simulink model "uz_ParameterID"  (R2021a)
settings: Solver=FixedStepDiscrete  StartTime=0.0  StopTime=160  FixedStep=0.000005  RelTol=1e-3  EnableMultiTasking=on
model workspace (MATLAB code in the model file):
  | cmdLim = Simulink.Parameter;
  | cmdLim.Value = 15;
  | cmdLim.Description = 'Limit for controlling the maximum surface command angle.';
  | cmdLim.Min = 0;
  | cmdLim.Max = 90;
  | cmdLim.DocUnits = 'deg';
  | 
  | dispGain = Simulink.Parameter;
  | dispGain.Value = 0.75;
  | dispGain.Description = 'Gain applied to the displacement error.';
  | dispGain.Min = 0;
  | dispGain.Max = [];
  | dispGain.DocUnits = 'deg/sec/deg';
  | 
  | dispLim = Simulink.Parameter;
  | dispLim.Value = 30;
  | dispLim.Description = 'Limit for controlling the maximum commanded angle.';
  | dispLim.Min = 0;
  | dispLim.Max = 180;
  | dispLim.DocUnits = 'deg';
  | 
  | intGain = Simulink.Parameter;
  | intGain.Value = 0.5;
  | intGain.Description = 'Gain applied to the integral error.';
  | intGain.Min = 0;
  | intGain.Max = [];
  | intGain.DocUnits = 'deg/sec/deg/sec';
  | 
  | intLim = Simulink.Parameter;
  | intLim.Value = 5;
  | intLim.Description = 'Limit for controlling the maximum commanded angle.';
  | intLim.Min = 0;
  | intLim.Max = 90;
  | intLim.DocUnits = 'deg';
  | 
  | rateGain = Simulink.Parameter;
  | rateGain.Value = 2;
  | rateGain.Description = 'Gain applied to the rate error.';
  | rateGain.Min = 0;
  | rateGain.Max = [];
  | rateGain.DocUnits = 'deg/deg/sec';
  | 
  | rateLim = Simulink.Parameter;
  | rateLim.Value = 6;
  | rateLim.Description = 'Limit for controlling the maximum commanded angle.';
  | rateLim.Min = 0;
  | rateLim.Max = 180;
  | rateLim.DocUnits = 'deg/sec';
  | 
  | hdgGain = Simulink.Parameter;
  | hdgGain.Value = 0.015;
values from neighbouring files (symbols this model uses):
  d_d_TMS = 0.005    [Parameter_Init_Buehler_201.m]
  d_f_hardware = 200000    [Parameter_Init_Buehler_201.m]
  d_f_states = 20000    [Parameter_Init_Buehler_201.m]
  d_i_max = 15    [Parameter_Init_Buehler_201.m]
  d_i_min = -d_i_max    (= -15)    [Parameter_Init_Buehler_201.m]
  d_I_n = 8    [Parameter_Init_Buehler_201.m]
  d_J_Coupling_M_E = 2e-6    (= 2e-06)    [Parameter_Init_Buehler_201.m]
  d_J_Coupling_M_Ms = 2e-20    [Parameter_Init_Buehler_201.m]
  d_J_Ms_L = d_J_Ms_M    (= 1.26363648e-05)    [Parameter_Init_Buehler_201.m]
  d_J_Ms_M = 0.5*0.5*((0.5*d_d_Ms)^4)*3.14*d_l_Ms*d_rho_Ms    (= 1.26363648e-05)    [Parameter_Init_Buehler_201.m]
  d_Ki_id = 162.47    [Parameter_Init_Buehler_201.m]
  d_Ki_iq = 162.47    [Parameter_Init_Buehler_201.m]
  d_Ki_n = 1.982    [Parameter_Init_Buehler_201.m]
  d_Kp_id = 0.369    [Parameter_Init_Buehler_201.m]
  d_Kp_iq = 0.369    [Parameter_Init_Buehler_201.m]
  d_Kp_n = 0.198    [Parameter_Init_Buehler_201.m]
  d_L_d = 0.00031    [Parameter_Init_Buehler_201.m]
  d_L_q = 0.00033    [Parameter_Init_Buehler_201.m]
  d_n_n = 3200    [Parameter_Init_Buehler_201.m]
  d_p = 4    [Parameter_Init_Buehler_201.m]
  d_psi_pm = 0.0075    [Parameter_Init_Buehler_201.m]
  d_R_ph = d_R_ph_ph/2    (= 0.089)    [Parameter_Init_Buehler_201.m]
  d_y_max = 10    [Parameter_Init_Buehler_201.m]
  d_y_min = -d_y_max    (= -10)    [Parameter_Init_Buehler_201.m]
undefined symbols (not defined in the file or in its folder): i_dq, i_dq_ref, n_ref, V_abc, v_dq
libraries: fl_lib x47, nesl_utility x30, ee_lib x18, simulink x8, spsabctodq0Lib x2, spsdq0toabcLib x1, spsTriangleGeneratorLib x1
(part 3 of 4)

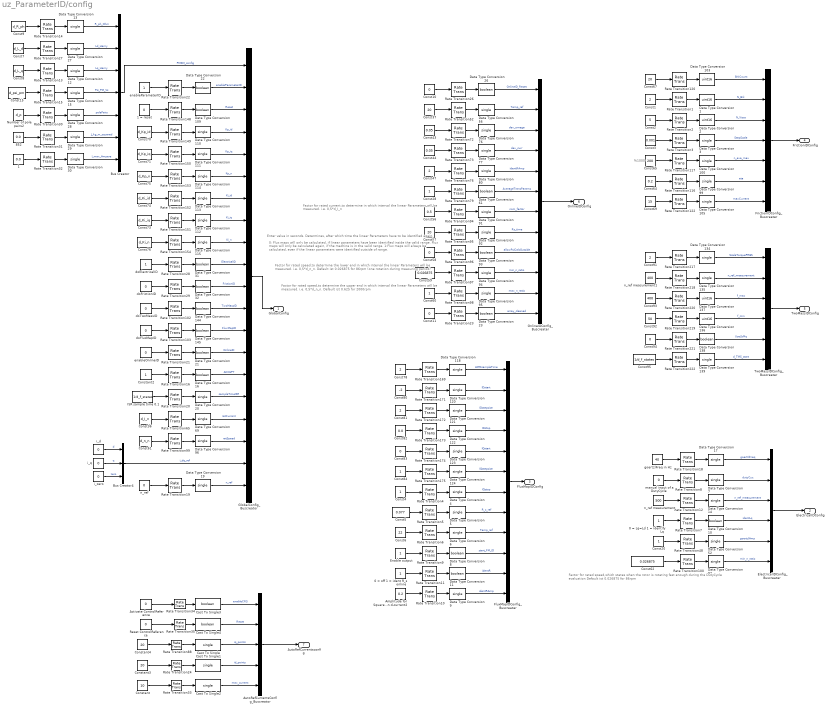
== system uz_ParameterID/config ==
  note: %1000
  note: Factor for rated speed,to determine the upper end in which interval the linear Parameters will
      | be measured. i.e. 0,5*d_n_n.
      | Default ist 0.625 for 2000rpm
  note: 0: Flux maps will only be calculated, if linear parameters have been identified inside the valid range.
      |     Flux maps will only be calculated again, if the machine is in the valid range.
      | 1:Flux maps will always be calculated, even if the linear parameters were identified outside of range.
  note: Enter value in seconds. Determines, after which time the linear Parameters have to be identified again.
  note: Factor for rated current,to determine in which interval the linear Parameters will
      | be measured. i.e. 0,5*d_I_n
  note: Factor for rated speed,to determine the lower end in which interval the linear Parameters will
      | be measured. i.e. 0,5*d_n_n.
      | Default ist 0.026875 for 86rpm (one rotation during measuring period)
  note: Factor for rated speed,which states when the rotor is rotating fast enough during the DutyCycle evaluation
      | Default ist 0.026875 for 86rpm
  "0 = Lq=Ld 1 = identify Lq " : Constant
  0 = off 1 = ident R_s online : Constant
  1 : Constant  Value=0.0
  1 = reset : Constant  Value=0
  852 : Constant  Value=0.0
  Activate ControlReference : Constant  Value=0  OutDataTypeStr=boolean
  Amplitude for SquareWave signal in d-current2 : Constant  Value=0.2
  AutoRefCurrentsConfig_Buscreator : BusCreator  Inputs=5  OutDataTypeStr=Bus: uz_ParaID_AutoRefCurrentsConfig_t
  Bus Creator : BusCreator  Inputs=7  OutDataTypeStr=Bus: uz_PMSM_t
  Bus Creator4 : BusCreator  Inputs=3  OutDataTypeStr=Bus: uz_3ph_dq_t
  Cast To Single : DataTypeConversion  OutDataTypeStr=single
  Cast To Single1 : DataTypeConversion  OutDataTypeStr=single
  Cast To Single2 : DataTypeConversion  OutDataTypeStr=single
  Cast To Single3 : DataTypeConversion  OutDataTypeStr=boolean
  Cast To Single4 : DataTypeConversion  OutDataTypeStr=boolean
  Const{1,47,78,81,91} (5 alike) : Constant  Value=2
  Const{10..11,58,83,94} (5 alike) : Constant  Value=0
  Const15 : Constant  Value=d_psi_pm
  Const2 : Constant  Value=5
  Const{4,20,28,60,84} (5 alike) : Constant
  Const3 : Constant  Value=0.001
  Const36 : Constant  Value=d_I_n
  Const37 : Constant  Value=20
  Const43 : Constant  Value=0.05
  Const44 : Constant  Value=0.05
  Const5 : Constant  Value=0.077
  Const56 : Constant  Value=0.5
  Const57 : Constant  Value=20
  Const59 : Constant  Value=0.026875
  Const6 : Constant  Value=22
  Const61 : Constant  Value=d_n_n
  Const62 : Constant  Value=0.026875
  Const64 : Constant  Value=0.2
  Const65 : Constant  Value=200
  Const67 : Constant  Value=20
  Const69 : Constant  Value=15
  Const7 : Constant  Value=d_L_d
  Const70 : Constant  Value=d_Kp_id
  Const71 : Constant  Value=d_Kp_iq
  Const73 : Constant  Value=d_Ki_iq
  Const74 : Constant  Value=d_Ki_id
  Const75 : Constant  Value=d_Kp_n
  Const76 : Constant  Value=d_Ki_n
  Const8 : Constant  Value=d_L_q
  Const80 : Constant  Value=-2
  Const82 : Constant  Value=0.0
  Const9 : Constant  Value=d_R_ph
  Const92 : Constant  Value=50
  Const93 : Constant  Value=400
  Const95 : Constant  Value=1/d_f_states
  Constant : Constant  Value=10
  Constant2 : Constant
  Constant3 : Constant  Value=20
  Constant4 : Constant  Value=20
  Data Type Conversion{1..2,103,136..137} (5 alike) : DataTypeConversion  OutDataTypeStr=uint16
  Data Type Conversion{8,10..11,16,21..23,26,31..32,61,93,109,138,144..145} (16 alike) : DataTypeConversion  OutDataTypeStr=boolean
  Data Type Conversion{3..7,9,12..15,17,19..20,27..30,52,56,69,76..77,80,91..92,94..97,99..100,105,110..115,118,120..124,134..135,139} (47 alike) : DataTypeConversion  OutDataTypeStr=single
  ElectricalIDConfig_Buscreater : BusCreator  Inputs=6  OutDataTypeStr=Bus: uz_ParaID_ElectricalIDConfig_t
  Enable output : Constant
  FluxMapIDConfig_Buscreater : BusCreator  Inputs=12  OutDataTypeStr=Bus: uz_ParaID_FluxMapIDConfig_t
  FrictionIDConfig_Buscreater : BusCreator  Inputs=7  OutDataTypeStr=Bus: uz_ParaID_FrictionIDConfig_t
  GlobalConfig_Buscreator : BusCreator  Inputs=20  OutDataTypeStr=Bus: uz_ParaID_GlobalConfig_t
  ISR sample time 0.1 : Constant  Value=1/d_f_states
  Number of pole pairs2 : Constant  Value=d_p
  OnlineIDConfig_Buscreater : BusCreator  Inputs=12  OutDataTypeStr=Bus: uz_ParaID_OnlineIDConfig_t
  Rate Transition{1..16,18..24,26..35,48,52,65,72..73,76,79,88,94..100,102..103,116..117,120,122,148..154,169,171..175,217..222} (73 alike) : RateTransition  OutPortSampleTime=1/d_f_states
  Reset ControlReference : Constant  Value=0  OutDataTypeStr=boolean
  TwoMassIDConfig_Buscreater : BusCreator  Inputs=6  OutDataTypeStr=Bus: uz_ParaID_TwoMassIDConfig_t
  doElectricalID : Constant
  doFluxMapID : Constant  Value=0
  doFrictionID : Constant  Value=0
  doTwoMassID : Constant  Value=0
  enableOnlineID : Constant  Value=0
  enableParameterID : Constant
  goertzlFreq in Hz : Constant  Value=40
  i_d : Constant  Value=0  OutDataTypeStr=single
  i_q : Constant  Value=0  OutDataTypeStr=single
  i_zero : Constant  Value=0  OutDataTypeStr=single
  manual input of a DutyCycle : Constant  Value=0
  n_ref : Constant  Value=0
  n_ref measurement : Constant  Value=500
  n_ref measurement1 : Constant  Value=400
  GlobalConfig : Outport
  ElectricalIDConfig : Outport  Port=2
  FluxMapIDConfig : Outport  Port=3
  FrictionIDConfig : Outport  Port=4
  TwoMassIDConfig : Outport  Port=5
  OnlineIDConfig : Outport  Port=6
  AutoRefCurrentsconfig : Outport  Port=7
  wires:
  Data Type Conversion1/1 -> FrictionIDConfig_Buscreater/2  "N_Brk"
  Data Type Conversion99/1 -> FrictionIDConfig_Buscreater/6  "eta"
  Data Type Conversion2/1 -> FrictionIDConfig_Buscreater/3  "N_Visco"
  Data Type Conversion103/1 -> FrictionIDConfig_Buscreater/1  "BrkCount"
  Data Type Conversion105/1 -> FrictionIDConfig_Buscreater/7  "maxCurrent"
  Data Type Conversion100/1 -> FrictionIDConfig_Buscreater/5  "n_eva_max"
  Data Type Conversion3/1 -> FrictionIDConfig_Buscreater/4  "StepScale"
  FrictionIDConfig_Buscreater/1 -> FrictionIDConfig/1
  Rate Transition120/1 -> Data Type Conversion103/1
  Const67/1 -> Rate Transition120/1
  Const1/1 -> Rate Transition1/1
  Rate Transition1/1 -> Data Type Conversion1/1
  Const2/1 -> Rate Transition2/1
  Rate Transition2/1 -> Data Type Conversion2/1
  Const3/1 -> Rate Transition3/1
  Rate Transition3/1 -> Data Type Conversion3/1
  Const65/1 -> Rate Transition117/1
  Const64/1 -> Rate Transition116/1
  Rate Transition116/1 -> Data Type Conversion99/1
  Rate Transition117/1 -> Data Type Conversion100/1
  Const69/1 -> Rate Transition122/1
  Rate Transition122/1 -> Data Type Conversion105/1
  TwoMassIDConfig_Buscreater/1 -> TwoMassIDConfig/1
  Const91/1 -> Rate Transition217/1
  Rate Transition217/1 -> Data Type Conversion134/1
  Data Type Conversion134/1 -> TwoMassIDConfig_Buscreater/1  "ScaleTorquePRBS"
  Rate Transition218/1 -> Data Type Conversion135/1
  n_ref measurement1/1 -> Rate Transition218/1
  Data Type Conversion135/1 -> TwoMassIDConfig_Buscreater/2  "n_ref_measurement"
  Rate Transition219/1 -> Data Type Conversion136/1
  Const93/1 -> Rate Transition220/1
  Const92/1 -> Rate Transition219/1
  Rate Transition220/1 -> Data Type Conversion137/1
  Data Type Conversion137/1 -> TwoMassIDConfig_Buscreater/3  "f_max"
  Data Type Conversion136/1 -> TwoMassIDConfig_Buscreater/4  "f_min"
  Rate Transition221/1 -> Data Type Conversion138/1
  Rate Transition222/1 -> Data Type Conversion139/1
  Const94/1 -> Rate Transition221/1
  Const95/1 -> Rate Transition222/1
  Data Type Conversion138/1 -> TwoMassIDConfig_Buscreater/5  "UseLbMq"
  Data Type Conversion139/1 -> TwoMassIDConfig_Buscreater/6  "d_TMS_start"
  FluxMapIDConfig_Buscreater/1 -> FluxMapIDConfig/1
  Rate Transition172/1 -> Data Type Conversion121/1
  Const80/1 -> Rate Transition171/1
  Const84/1 -> Rate Transition175/1
  Rate Transition175/1 -> Data Type Conversion124/1
  Rate Transition171/1 -> Data Type Conversion120/1
  Rate Transition174/1 -> Data Type Conversion123/1
  Const78/1 -> Rate Transition169/1
  Const82/1 -> Rate Transition173/1
  Const81/1 -> Rate Transition172/1
  Rate Transition169/1 -> Data Type Conversion118/1
  Rate Transition173/1 -> Data Type Conversion122/1
  Const83/1 -> Rate Transition174/1
  Data Type Conversion118/1 -> FluxMapIDConfig_Buscreater/1  "AMMsampleTime"
  Data Type Conversion120/1 -> FluxMapIDConfig_Buscreater/2  "IDstart"
  Rate Transition5/1 -> Data Type Conversion5/1
  Rate Transition6/1 -> Data Type Conversion6/1
  Const6/1 -> Rate Transition6/1
  Const4/1 -> Rate Transition4/1
  Const5/1 -> Rate Transition5/1
  Rate Transition4/1 -> Data Type Conversion4/1
  Data Type Conversion121/1 -> FluxMapIDConfig_Buscreater/3  "IDstepsize"
  Data Type Conversion122/1 -> FluxMapIDConfig_Buscreater/4  "IDstop"
  Data Type Conversion123/1 -> FluxMapIDConfig_Buscreater/5  "IQstart"
  Data Type Conversion124/1 -> FluxMapIDConfig_Buscreater/6  "IQstepsize"
  Data Type Conversion4/1 -> FluxMapIDConfig_Buscreater/7  "IQstop"
  Data Type Conversion5/1 -> FluxMapIDConfig_Buscreater/8  "R_s_ref"
  Data Type Conversion6/1 -> FluxMapIDConfig_Buscreater/9  "Temp_ref"
  ElectricalIDConfig_Buscreater/1 -> ElectricalIDConfig/1
  OnlineIDConfig_Buscreater/1 -> OnlineIDConfig/1
  Const37/1 -> Rate Transition52/1
  Rate Transition52/1 -> Data Type Conversion56/1
  Data Type Conversion56/1 -> OnlineIDConfig_Buscreater/2  "Temp_ref"
  Data Type Conversion77/1 -> OnlineIDConfig_Buscreater/4  "dev_curr"
  Data Type Conversion76/1 -> OnlineIDConfig_Buscreater/3  "dev_omega"
  Const44/1 -> Rate Transition73/1
  Const43/1 -> Rate Transition72/1
  Rate Transition72/1 -> Data Type Conversion76/1
  Const47/1 -> Rate Transition76/1
  Rate Transition73/1 -> Data Type Conversion77/1
  Rate Transition76/1 -> Data Type Conversion80/1
  Data Type Conversion80/1 -> OnlineIDConfig_Buscreater/5  "identRAmp"
  Data Type Conversion61/1 -> OnlineIDConfig_Buscreater/6  "AverageTransParams"
  Const28/1 -> Rate Transition79/1
  Rate Transition79/1 -> Data Type Conversion61/1
  Const56/1 -> Rate Transition94/1
  Data Type Conversion93/1 -> OnlineIDConfig_Buscreater/9  "allowPsiCalcOutside"
  Rate Transition94/1 -> Data Type Conversion91/1
  Data Type Conversion95/1 -> OnlineIDConfig_Buscreater/11  "max_n_ratio"
  Const58/1 -> Rate Transition96/1
  Const57/1 -> Rate Transition95/1
  Data Type Conversion91/1 -> OnlineIDConfig_Buscreater/7  "nom_factor"
  Rate Transition98/1 -> Data Type Conversion95/1
  Data Type Conversion92/1 -> OnlineIDConfig_Buscreater/8  "Rs_time"
  Rate Transition96/1 -> Data Type Conversion93/1
  Const59/1 -> Rate Transition97/1
  Rate Transition97/1 -> Data Type Conversion94/1
  Const60/1 -> Rate Transition98/1
  Data Type Conversion94/1 -> OnlineIDConfig_Buscreater/10  "min_n_ratio"
  Rate Transition95/1 -> Data Type Conversion92/1
  1 = reset/1 -> Rate Transition148/1
  Rate Transition149/1 -> Data Type Conversion110/1
  Const75/1 -> Rate Transition153/1
  Rate Transition150/1 -> Data Type Conversion111/1
  Rate Transition152/1 -> Data Type Conversion113/1
  Const71/1 -> Rate Transition150/1
  Rate Transition154/1 -> Data Type Conversion115/1
  Const76/1 -> Rate Transition154/1
  Rate Transition148/1 -> Data Type Conversion109/1
  Const70/1 -> Rate Transition149/1
  Rate Transition153/1 -> Data Type Conversion114/1
  Const73/1 -> Rate Transition151/1
  Rate Transition151/1 -> Data Type Conversion112/1
  Const74/1 -> Rate Transition152/1
  Data Type Conversion109/1 -> GlobalConfig_Buscreator/3  "Reset"
  Data Type Conversion110/1 -> GlobalConfig_Buscreator/4  "Kp_id"
  Data Type Conversion111/1 -> GlobalConfig_Buscreator/5  "Kp_iq"
  Data Type Conversion114/1 -> GlobalConfig_Buscreator/6  "Kp_n"
  Data Type Conversion113/1 -> GlobalConfig_Buscreator/7  "Ki_id"
  Data Type Conversion112/1 -> GlobalConfig_Buscreator/8  "Ki_iq"
  Data Type Conversion115/1 -> GlobalConfig_Buscreator/9  "Ki_n"
  Rate Transition28/1 -> Data Type Conversion31/1
  Data Type Conversion32/1 -> GlobalConfig_Buscreator/11  "FrictionID"
  doTwoMassID/1 -> Rate Transition102/1
  Data Type Conversion145/1 -> GlobalConfig_Buscreator/13  "FluxMapID"
  Rate Transition29/1 -> Data Type Conversion32/1
  doFluxMapID/1 -> Rate Transition103/1
  Rate Transition103/1 -> Data Type Conversion145/1
  Data Type Conversion31/1 -> GlobalConfig_Buscreator/10  "ElectricalID"
  Rate Transition102/1 -> Data Type Conversion144/1
  doElectricalID/1 -> Rate Transition28/1
  Data Type Conversion144/1 -> GlobalConfig_Buscreator/12  "TwoMassID"
  doFrictionID/1 -> Rate Transition29/1
  Constant2/1 -> Rate Transition16/1
  Rate Transition16/1 -> Data Type Conversion16/1
  Data Type Conversion16/1 -> GlobalConfig_Buscreator/15  "ACCEPT"
  ISR sample time 0.1/1 -> Rate Transition20/1
  Rate Transition20/1 -> Data Type Conversion20/1
  Const36/1 -> Rate Transition65/1
  Const61/1 -> Rate Transition99/1
  Rate Transition99/1 -> Data Type Conversion96/1
  Rate Transition65/1 -> Data Type Conversion69/1
  Data Type Conversion69/1 -> GlobalConfig_Buscreator/17  "ratCurrent"
  Data Type Conversion96/1 -> GlobalConfig_Buscreator/18  "ratSpeed"
  enableOnlineID/1 -> Rate Transition21/1
  Data Type Conversion21/1 -> GlobalConfig_Buscreator/14  "OnlineID"
  Rate Transition21/1 -> Data Type Conversion21/1
  GlobalConfig_Buscreator/1 -> GlobalConfig/1
  Rate Transition26/1 -> Data Type Conversion26/1
  Data Type Conversion26/1 -> OnlineIDConfig_Buscreater/1  "OnlineID_Reset"
  Const10/1 -> Rate Transition26/1
  Data Type Conversion11/1 -> FluxMapIDConfig_Buscreater/11  "identR"
  0 = off 1 = ident R_s online/1 -> Rate Transition11/1
  Rate Transition10/1 -> Data Type Conversion9/1
  Amplitude for SquareWave signal in d-current2/1 -> Rate Transition10/1
  Data Type Conversion9/1 -> FluxMapIDConfig_Buscreater/12  "identRAmp"
  Rate Transition11/1 -> Data Type Conversion11/1
  Data Type Conversion8/1 -> FluxMapIDConfig_Buscreater/10  "start_FM_ID"
  Rate Transition9/1 -> Data Type Conversion8/1
  Enable output/1 -> Rate Transition9/1
  Bus Creator/1 -> GlobalConfig_Buscreator/1  "PMSM_config"
  Const15/1 -> Rate Transition15/1
  Rate Transition15/1 -> Data Type Conversion15/1
  Data Type Conversion15/1 -> Bus Creator/4  "Psi_PM_Vs"
  Rate Transition30/1 -> Data Type Conversion28/1
  Number of pole pairs2/1 -> Rate Transition30/1
  Data Type Conversion28/1 -> Bus Creator/5  "polePairs"
  Rate Transition31/1 -> Data Type Conversion29/1
  852/1 -> Rate Transition31/1
  Data Type Conversion29/1 -> Bus Creator/6  "J_kg_m_squared"
  Rate Transition32/1 -> Data Type Conversion30/1
  1/1 -> Rate Transition32/1
  Data Type Conversion30/1 -> Bus Creator/7  "I_max_Ampere"
  Data Type Conversion13/1 -> Bus Creator/1  "R_ph_Ohm"
  Const9/1 -> Rate Transition14/1
  Rate Transition14/1 -> Data Type Conversion13/1
  Data Type Conversion27/1 -> Bus Creator/2  "Ld_Henry"
  Rate Transition13/1 -> Data Type Conversion12/1
  Rate Transition27/1 -> Data Type Conversion27/1
  Data Type Conversion12/1 -> Bus Creator/3  "Lq_Henry"
  Const7/1 -> Rate Transition27/1
  Const8/1 -> Rate Transition13/1
  i_q/1 -> Bus Creator4/2  "q"
  i_d/1 -> Bus Creator4/1  "d"
  i_zero/1 -> Bus Creator4/3  "zero"
  Bus Creator4/1 -> GlobalConfig_Buscreator/19  "i_dq_ref"
  Rate Transition19/1 -> Data Type Conversion19/1
  n_ref/1 -> Rate Transition19/1
  Data Type Conversion19/1 -> GlobalConfig_Buscreator/20  "n_ref"
  enableParameterID/1 -> Rate Transition22/1
  Rate Transition22/1 -> Data Type Conversion22/1
  Data Type Conversion22/1 -> GlobalConfig_Buscreator/2  "enableParameterID"
  Rate Transition23/1 -> Data Type Conversion23/1
  Const11/1 -> Rate Transition23/1
  Data Type Conversion23/1 -> OnlineIDConfig_Buscreater/12  "array_cleaned"
  Constant4/1 -> Rate Transition88/1
  Rate Transition88/1 -> Cast To Single/1
  Rate Transition24/1 -> Cast To Single1/1
  Constant3/1 -> Rate Transition24/1
  Rate Transition33/1 -> Cast To Single2/1
  Constant/1 -> Rate Transition33/1
  Rate Transition34/1 -> Cast To Single3/1
  Cast To Single3/1 -> AutoRefCurrentsConfig_Buscreator/1  "enableCRS"
  Activate ControlReference/1 -> Rate Transition34/1
  Rate Transition35/1 -> Cast To Single4/1
  Reset ControlReference/1 -> Rate Transition35/1
  Cast To Single4/1 -> AutoRefCurrentsConfig_Buscreator/2  "Reset"
  Cast To Single/1 -> AutoRefCurrentsConfig_Buscreator/3  "iq_points"
  Cast To Single1/1 -> AutoRefCurrentsConfig_Buscreator/4  "id_points"
  Cast To Single2/1 -> AutoRefCurrentsConfig_Buscreator/5  "max_current"
  AutoRefCurrentsConfig_Buscreator/1 -> AutoRefCurrentsconfig/1
  Data Type Conversion20/1 -> GlobalConfig_Buscreator/16  "sampleTimeISR"
  Rate Transition18/1 -> Data Type Conversion17/1
  Data Type Conversion17/1 -> ElectricalIDConfig_Buscreater/1  "goertzlFreq"
  goertzlFreq in Hz/1 -> Rate Transition18/1
  Rate Transition8/1 -> Data Type Conversion7/1
  Const20/1 -> Rate Transition48/1
  Data Type Conversion14/1 -> ElectricalIDConfig_Buscreater/3  "n_ref_measurement"
  manual input of a DutyCycle/1 -> Rate Transition8/1
  "0 = Lq=Ld 1 = identify Lq "/1 -> Rate Transition7/1
  Const62/1 -> Rate Transition100/1
  n_ref measurement/1 -> Rate Transition12/1
  Data Type Conversion7/1 -> ElectricalIDConfig_Buscreater/2  "dutyCyc"
  Data Type Conversion97/1 -> ElectricalIDConfig_Buscreater/6  "min_n_ratio"
  Rate Transition7/1 -> Data Type Conversion10/1
  Rate Transition48/1 -> Data Type Conversion52/1
  Rate Transition12/1 -> Data Type Conversion14/1
  Data Type Conversion52/1 -> ElectricalIDConfig_Buscreater/5  "goertzlAmp"
  Data Type Conversion10/1 -> ElectricalIDConfig_Buscreater/4  "identLq"
  Rate Transition100/1 -> Data Type Conversion97/1

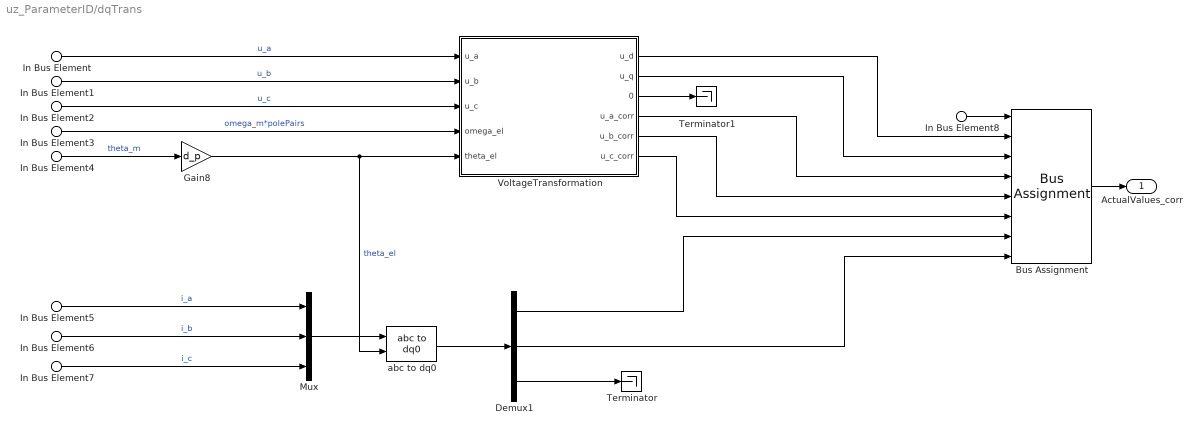
== system uz_ParameterID/dqTrans ==
  In Bus Element8 : Inport  PortName=ActualValues
  In Bus Element3 : Inport  PortName=ActualValues  Element=omega_el
  In Bus Element4 : Inport  PortName=ActualValues  Element=theta_m
  In Bus Element : Inport  PortName=ActualValues  Element=V_abc.a
  In Bus Element1 : Inport  PortName=ActualValues  Element=V_abc.b
  In Bus Element2 : Inport  PortName=ActualValues  Element=V_abc.c
  In Bus Element5 : Inport  PortName=ActualValues  Element=I_abc.a
  In Bus Element6 : Inport  PortName=ActualValues  Element=I_abc.b
  In Bus Element7 : Inport  PortName=ActualValues  Element=I_abc.c
  Bus Assignment : BusAssignment  AssignedSignals=v_dq.d,v_dq.q,V_abc.a,V_abc.b,V_abc.c,i_dq.d,i_dq.q
  Demux1 : Demux  Outputs=3
  Gain8 : Gain  Gain=d_p  OutDataTypeStr=single
  Mux : Mux  Inputs=3
  Terminator : Terminator
  Terminator1 : Terminator
  VoltageTransformation : Subsystem
  abc to dq0 : spsabctodq0Lib/abc to dq0  Alignment=Aligned with phase A axis
  ActualValues_corr : Outport  OutDataTypeStr=Bus: uz_ParaID_ActualValues_t
  wires:
  VoltageTransformation/3(0) -> Terminator1/1
  In Bus Element3/1 -> VoltageTransformation/4(omega_el)  "omega_m*polePairs"
  In Bus Element2/1 -> VoltageTransformation/3(u_c)  "u_c"
  In Bus Element1/1 -> VoltageTransformation/2(u_b)  "u_b"
  In Bus Element/1 -> VoltageTransformation/1(u_a)  "u_a"
  Demux1/3 -> Terminator/1
  Mux/1 -> abc to dq0/1
  In Bus Element7/1 -> Mux/3  "i_c"
  In Bus Element6/1 -> Mux/2  "i_b"
  In Bus Element5/1 -> Mux/1  "i_a"
  Demux1/2 -> Bus Assignment/8
  Demux1/1 -> Bus Assignment/7
  abc to dq0/1 -> Demux1/1
  VoltageTransformation/2(u_q) -> Bus Assignment/3
  VoltageTransformation/1(u_d) -> Bus Assignment/2
  VoltageTransformation/4(u_a_corr) -> Bus Assignment/4
  VoltageTransformation/5(u_b_corr) -> Bus Assignment/5
  VoltageTransformation/6(u_c_corr) -> Bus Assignment/6
  In Bus Element8/1 -> Bus Assignment/1
  Bus Assignment/1 -> ActualValues_corr/1
  Gain8/1 -> abc to dq0/2, VoltageTransformation/5(theta_el)  "theta_el"
  In Bus Element4/1 -> Gain8/1  "theta_m"

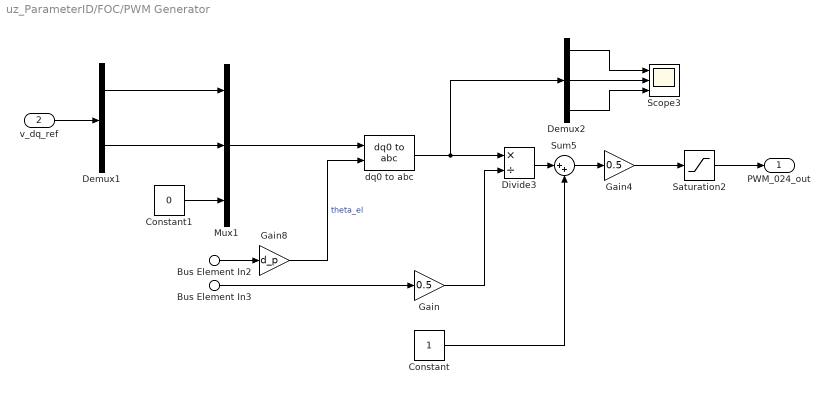
== system uz_ParameterID/FOC/PWM Generator ==
  Bus Element In2 : Inport  PortName=ActualValues  Element=theta_m
  Bus Element In3 : Inport  PortName=ActualValues  Element=V_DC
  v_dq_ref : Inport  Port=2
  Constant : Constant  OutDataTypeStr=single
  Constant1 : Constant  Value=0  OutDataTypeStr=single
  Demux1 : Demux  Outputs=2
  Demux2 : Demux  Outputs=3
  Divide3 : Product  Inputs=*/
  Gain : Gain  Gain=0.5
  Gain4 : Gain  Gain=0.5
  Gain8 : Gain  Gain=d_p  OutDataTypeStr=single
  Mux1 : Mux  Inputs=3
  Saturation2 : Saturate  UpperLimit=1  LowerLimit=0
  Scope3 : Scope  NumInputPorts=3
  Sum5 : Sum  Inputs=|++
  dq0 to abc : spsdq0toabcLib/dq0 to abc  Alignment=Aligned with phase A axis
  PWM_024_out : Outport  VectorParamsAs1DForOutWhenUnconnected=off
  wires:
  Constant/1 -> Sum5/2
  Demux2/2 -> Scope3/2
  Gain4/1 -> Saturation2/1
  Demux2/1 -> Scope3/1
  Demux2/3 -> Scope3/3
  Gain/1 -> Divide3/2
  Sum5/1 -> Gain4/1
  Mux1/1 -> dq0 to abc/1
  dq0 to abc/1 -> Demux2/1, Divide3/1
  Divide3/1 -> Sum5/1
  Bus Element In3/1 -> Gain/1
  Constant1/1 -> Mux1/3
  Demux1/2 -> Mux1/2
  Saturation2/1 -> PWM_024_out/1
  v_dq_ref/1 -> Demux1/1
  Demux1/1 -> Mux1/1
  Bus Element In2/1 -> Gain8/1
  Gain8/1 -> dq0 to abc/2  "theta_el"

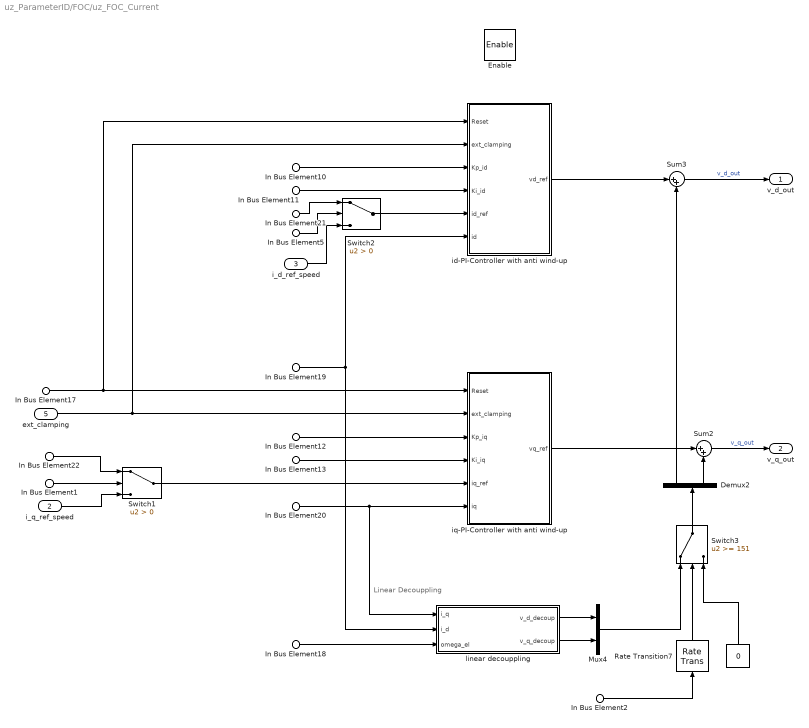
== system uz_ParameterID/FOC/uz_FOC_Current ==
  note: Linear Decouppling
  In Bus Element18 : Inport  PortName=ActualValues  Element=omega_el
  In Bus Element19 : Inport  PortName=ActualValues  Element=i_dq.d
  In Bus Element20 : Inport  PortName=ActualValues  Element=i_dq.q
  i_q_ref_speed : Inport  Port=2
  i_d_ref_speed : Inport  Port=3
  In Bus Element17 : Inport  Port=4  PortName=FOC_State_outputs  Element=resetIntegrator
  In Bus Element11 : Inport  Port=4  PortName=FOC_State_outputs  Element=Ki_id_out
  In Bus Element10 : Inport  Port=4  PortName=FOC_State_outputs  Element=Kp_id_out
  In Bus Element12 : Inport  Port=4  PortName=FOC_State_outputs  Element=Kp_iq_out
  In Bus Element13 : Inport  Port=4  PortName=FOC_State_outputs  Element=Ki_iq_out
  In Bus Element1 : Inport  Port=4  PortName=FOC_State_outputs  Element=enableFOC_current
  In Bus Element5 : Inport  Port=4  PortName=FOC_State_outputs  Element=enableFOC_current
  In Bus Element2 : Inport  Port=4  PortName=FOC_State_outputs  Element=activeState
  In Bus Element21 : Inport  Port=4  PortName=FOC_State_outputs  Element=i_dq_ref.d
  In Bus Element22 : Inport  Port=4  PortName=FOC_State_outputs  Element=i_dq_ref.q
  ext_clamping : Inport  Port=5
  Enable : EnablePort
  " " : Constant  Value=0  OutDataTypeStr=single
  Demux2 : Demux  Outputs=2
  Mux4 : Mux  Inputs=2
  Rate Transition7 : RateTransition  OutPortSampleTime=1/d_f_hardware
  Sum2 : Sum  Inputs=|++
  Sum3 : Sum  Inputs=|++
  Switch1 : Switch  Criteria=u2 > Threshold
  Switch2 : Switch  Criteria=u2 > Threshold
  Switch3 : Switch  Threshold=151
  id-PI-Controller with anti wind-up : Subsystem
  iq-PI-Controller with anti wind-up : Subsystem
  linear decouppling : Subsystem
  v_d_out : Outport
  v_q_out : Outport  Port=2
  wires:
  In Bus Element22/1 -> Switch1/1
  In Bus Element1/1 -> Switch1/2
  Demux2/2 -> Sum2/2
  id-PI-Controller with anti wind-up/1(vd_ref) -> Sum3/1
  In Bus Element19/1 -> id-PI-Controller with anti wind-up/6(id), linear decouppling/2(i_d)
  Demux2/1 -> Sum3/2
  linear decouppling/2(v_q_decoup) -> Mux4/2
  linear decouppling/1(v_d_decoup) -> Mux4/1
  ext_clamping/1 -> iq-PI-Controller with anti wind-up/2(ext_clamping), id-PI-Controller with anti wind-up/2(ext_clamping)
  Switch1/1 -> iq-PI-Controller with anti wind-up/5(iq_ref)
  Sum3/1 -> v_d_out/1  "v_d_out"
  In Bus Element10/1 -> id-PI-Controller with anti wind-up/3(Kp_id)
  In Bus Element18/1 -> linear decouppling/3(omega_el)
  In Bus Element17/1 -> iq-PI-Controller with anti wind-up/1(Reset), id-PI-Controller with anti wind-up/1(Reset)
  In Bus Element12/1 -> iq-PI-Controller with anti wind-up/3(Kp_iq)
  i_q_ref_speed/1 -> Switch1/3
  iq-PI-Controller with anti wind-up/1(vq_ref) -> Sum2/1
  In Bus Element20/1 -> linear decouppling/1(i_q), iq-PI-Controller with anti wind-up/6(iq)
  i_d_ref_speed/1 -> Switch2/3
  In Bus Element21/1 -> Switch2/1
  Switch2/1 -> id-PI-Controller with anti wind-up/5(id_ref)
  In Bus Element5/1 -> Switch2/2
  Mux4/1 -> Switch3/1
  In Bus Element13/1 -> iq-PI-Controller with anti wind-up/4(Ki_iq)
  In Bus Element11/1 -> id-PI-Controller with anti wind-up/4(Ki_id)
  Sum2/1 -> v_q_out/1  "v_q_out"
  In Bus Element2/1 -> Rate Transition7/1
  Rate Transition7/1 -> Switch3/2
  Switch3/1 -> Demux2/1
  " "/1 -> Switch3/3

== system uz_ParameterID/FOC/uz_FOC_Speed ==
  In Bus Element18 : Inport  PortName=ActualValues  Element=omega_el
  In Bus Element19 : Inport  PortName=ActualValues  Element=V_DC
  In Bus Element : Inport  Port=2  PortName=TwoMassID_output  Element=PRBS_out
  In Bus Element13 : Inport  Port=3  PortName=FOC_State_outputs  Element=Kp_n_out
  In Bus Element14 : Inport  Port=3  PortName=FOC_State_outputs  Element=Ki_n_out
  In Bus Element15 : Inport  Port=3  PortName=FOC_State_outputs  Element=n_ref_FOC
  In Bus Element5 : Inport  Port=3  PortName=FOC_State_outputs  Element=resetIntegrator
  In Bus Element21 : Inport  Port=3  PortName=FOC_State_outputs  Element=i_dq_ref.d
  ext_clamping : Inport  Port=4
  Enable : EnablePort
  Field Weakening : Subsystem
  Sum5 : Sum  Inputs=|++
  omega-PI-Controller with anti wind-up : Subsystem
  i_q_ref : Outport  OutDataTypeStr=single
  id_soll : Outport  Port=2  OutDataTypeStr=single
  wires:
  In Bus Element/1 -> Sum5/2  "PRBS Excitation"
  In Bus Element21/1 -> Field Weakening/3(id_ref_input)
  In Bus Element13/1 -> omega-PI-Controller with anti wind-up/3(Kp_n)
  Field Weakening/2(id_Soll) -> id_soll/1
  In Bus Element19/1 -> Field Weakening/2(V_DC)
  ext_clamping/1 -> omega-PI-Controller with anti wind-up/2(ext_clamping)
  In Bus Element18/1 -> Field Weakening/1(omega_el), omega-PI-Controller with anti wind-up/6(omega)
  In Bus Element14/1 -> omega-PI-Controller with anti wind-up/4(Ki_n)
  In Bus Element15/1 -> omega-PI-Controller with anti wind-up/5(n_ref_rpm)
  In Bus Element5/1 -> omega-PI-Controller with anti wind-up/1(Reset)
  omega-PI-Controller with anti wind-up/1(iq_ref) -> Sum5/1
  Sum5/1 -> i_q_ref/1
  Field Weakening/1(iq_max) -> omega-PI-Controller with anti wind-up/7(iq_max)

== system uz_ParameterID/Hardware/Coupling Encoder ==
  note: 1) Add Subsystem or Model blocks as valid variant choices.
      | 2) You cannot connect blocks at this level. At simulation, connectivity is automatically
      | determined, based on the active variant and port name matching.
  Inertia : Subsystem  VariantControl=(default)
  Spring Damper System : Subsystem  VariantControl=TMS1
  Input : PMIOPort  Side=Left
  output : PMIOPort  Port=2  Side=Right

== system uz_ParameterID/Hardware/Measurement Shaft ==
  note: 1) Add Subsystem or Model blocks as valid variant choices.
      | 2) You cannot connect blocks at this level. At simulation, connectivity is automatically
      | determined, based on the active variant and port name matching.
  Spring Damper System : Subsystem  VariantControl=TMS1
  default : Subsystem  VariantControl=(default)
  Input : PMIOPort  Side=Left
  output : PMIOPort  Port=2  Side=Right

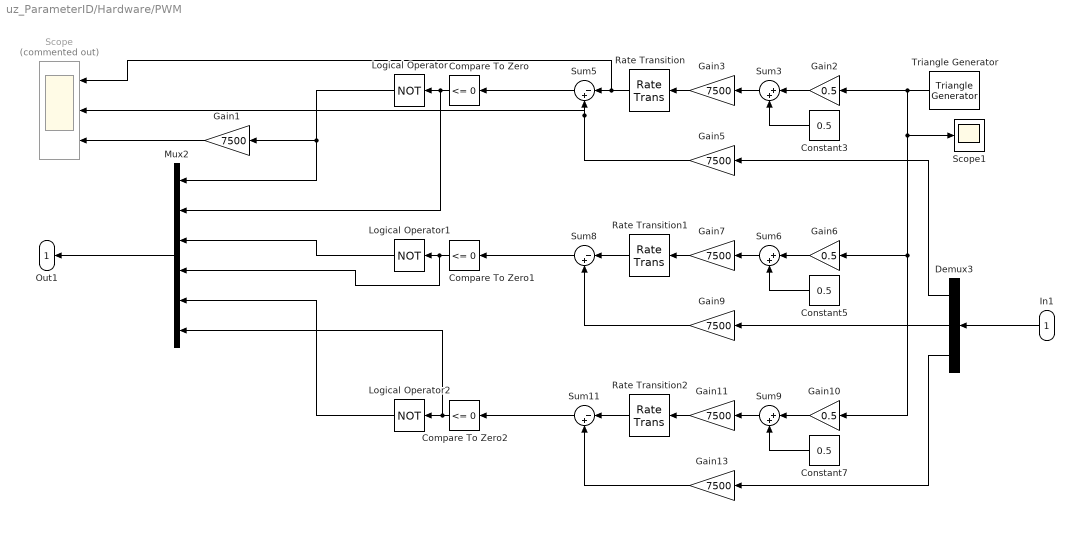
== system uz_ParameterID/Hardware/PWM ==
  In1 : Inport
  Compare To Zero : simulink/Logic and Bit Operations/Compare To Zero  relop=<=  OutDataTypeStr=boolean
  Compare To Zero1 : simulink/Logic and Bit Operations/Compare To Zero  relop=<=  OutDataTypeStr=boolean
  Compare To Zero2 : simulink/Logic and Bit Operations/Compare To Zero  relop=<=  OutDataTypeStr=boolean
  Constant3 : Constant  Value=0.5
  Constant5 : Constant  Value=0.5
  Constant7 : Constant  Value=0.5
  Demux3 : Demux  Outputs=3
  Gain{1,3,5,7,9,11,13} (7 alike) : Gain  Gain=7500  ParamDataTypeStr=single
  Gain10 : Gain  Gain=0.5
  Gain2 : Gain  Gain=0.5
  Gain6 : Gain  Gain=0.5
  Logical Operator : Logic  Operator=NOT  AllPortsSameDT=off  OutDataTypeStr=boolean
  Logical Operator1 : Logic  Operator=NOT  AllPortsSameDT=off  OutDataTypeStr=boolean
  Logical Operator2 : Logic  Operator=NOT  AllPortsSameDT=off  OutDataTypeStr=boolean
  Mux2 : Mux  Inputs=6
  Rate Transition : RateTransition  OutPortSampleTime=1/d_f_hardware
  Rate Transition1 : RateTransition  OutPortSampleTime=1/d_f_hardware
  Rate Transition2 : RateTransition  OutPortSampleTime=1/d_f_hardware
  Scope : Scope  Commented=on  NumInputPorts=3
  Scope1 : Scope
  Sum11 : Sum  Inputs=|-+
  Sum3 : Sum  Inputs=|++
  Sum5 : Sum  Inputs=|-+
  Sum6 : Sum  Inputs=|++
  Sum8 : Sum  Inputs=|-+
  Sum9 : Sum  Inputs=|++
  Triangle Generator : spsTriangleGeneratorLib/Triangle Generator  Freq=10000  Phase=0  Ts=0
  Out1 : Outport  VectorParamsAs1DForOutWhenUnconnected=off
  wires:
  Demux3/3 -> Gain13/1
  Logical Operator2/1 -> Mux2/5
  Logical Operator1/1 -> Mux2/3
  Mux2/1 -> Out1/1
  Compare To Zero2/1 -> Mux2/6, Logical Operator2/1
  Gain10/1 -> Sum9/1
  Sum8/1 -> Compare To Zero1/1
  Gain6/1 -> Sum6/1
  Sum9/1 -> Gain11/1
  Triangle Generator/1 -> Scope1/1, Gain10/1, Gain6/1, Gain2/1
  Sum6/1 -> Gain7/1
  Demux3/2 -> Gain9/1
  Compare To Zero1/1 -> Mux2/4, Logical Operator1/1
  Constant5/1 -> Sum6/2
  Constant7/1 -> Sum9/2
  Sum11/1 -> Compare To Zero2/1
  Sum3/1 -> Gain3/1
  Constant3/1 -> Sum3/2
  Demux3/1 -> Gain5/1
  Sum5/1 -> Compare To Zero/1
  Gain2/1 -> Sum3/1
  In1/1 -> Demux3/1
  Gain3/1 -> Rate Transition/1
  Gain7/1 -> Rate Transition1/1
  Gain11/1 -> Rate Transition2/1
  Gain5/1 -> Scope/2, Sum5/2
  Gain9/1 -> Sum8/2
  Gain13/1 -> Sum11/2
  Rate Transition/1 -> Scope/1, Sum5/1
  Rate Transition1/1 -> Sum8/1
  Rate Transition2/1 -> Sum11/1
  Logical Operator/1 -> Gain1/1, Mux2/1
  Compare To Zero/1 -> Mux2/2, Logical Operator/1
  Gain1/1 -> Scope/3

== system uz_ParameterID/Hardware/Switch f. TMS ==
  note: 1) Add Subsystem or Model blocks as valid variant choices.
      | 2) You cannot connect blocks at this level. At simulation, connectivity is automatically
      | determined, based on the active variant and port name matching.
  closed : Subsystem  VariantControl=d_KupplZus==1
  open : Subsystem  VariantControl=d_KupplZus==0
  Input : PMIOPort  Side=Left
  output : PMIOPort  Port=2  Side=Right

== system uz_ParameterID/Hardware/coupling m. shaft ==
  note: 1) Add Subsystem or Model blocks as valid variant choices.
      | 2) You cannot connect blocks at this level. At simulation, connectivity is automatically
      | determined, based on the active variant and port name matching.
  Inertia : Subsystem  VariantControl=(default)
  Spring Damper System : Subsystem  VariantControl=TMS1
  Input : PMIOPort  Side=Left
  output : PMIOPort  Port=2  Side=Right

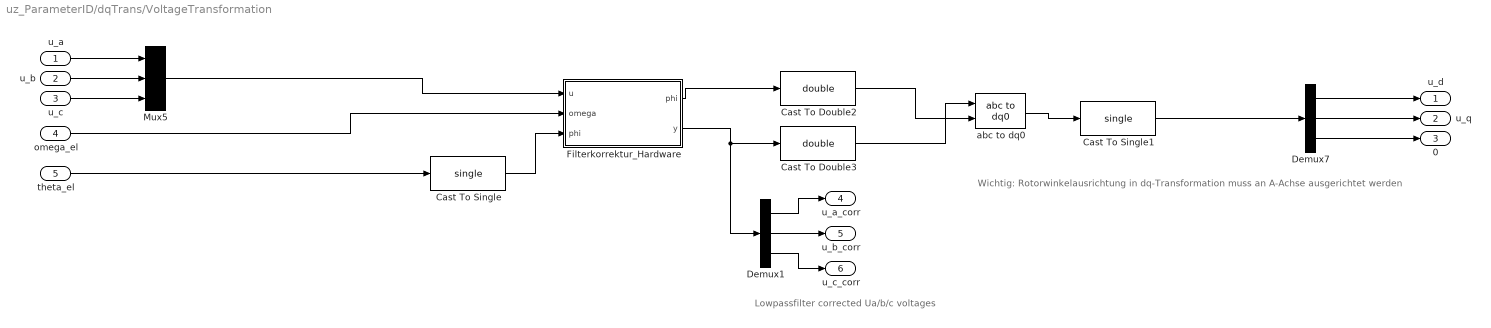
== system uz_ParameterID/dqTrans/VoltageTransformation ==
  note: Lowpassfilter corrected Ua/b/c voltages
  note: Wichtig: Rotorwinkelausrichtung in dq-Transformation
      | muss an A-Achse ausgerichtet werden
  u_a : Inport
  u_b : Inport  Port=2
  u_c : Inport  Port=3
  omega_el : Inport  Port=4
  theta_el : Inport  Port=5
  Cast To Double2 : DataTypeConversion  OutDataTypeStr=double
  Cast To Double3 : DataTypeConversion  OutDataTypeStr=double
  Cast To Single : DataTypeConversion  OutDataTypeStr=single
  Cast To Single1 : DataTypeConversion  OutDataTypeStr=single
  Demux1 : Demux  Outputs=3
  Demux7 : Demux  Outputs=3
  Filterkorrektur_Hardware : MATLAB Function  TreatAsAtomicUnit=on
  Mux5 : Mux  Inputs=3
  abc to dq0 : spsabctodq0Lib/abc to dq0  Alignment=Aligned with phase A axis
  u_d : Outport  VectorParamsAs1DForOutWhenUnconnected=off
  u_q : Outport  Port=2  VectorParamsAs1DForOutWhenUnconnected=off
  0 : Outport  Port=3  VectorParamsAs1DForOutWhenUnconnected=off
  u_a_corr : Outport  Port=4  VectorParamsAs1DForOutWhenUnconnected=off
  u_b_corr : Outport  Port=5  VectorParamsAs1DForOutWhenUnconnected=off
  u_c_corr : Outport  Port=6  VectorParamsAs1DForOutWhenUnconnected=off
  wires:
  abc to dq0/1 -> Cast To Single1/1
  Cast To Single1/1 -> Demux7/1
  Cast To Double3/1 -> abc to dq0/1
  Filterkorrektur_Hardware/2(y) -> Demux1/1, Cast To Double3/1
  Cast To Double2/1 -> abc to dq0/2
  Filterkorrektur_Hardware/1(phi) -> Cast To Double2/1
  Demux7/2 -> u_q/1
  Demux7/3 -> 0/1
  u_b/1 -> Mux5/2
  u_c/1 -> Mux5/3
  u_a/1 -> Mux5/1
  omega_el/1 -> Filterkorrektur_Hardware/2(omega)
  Mux5/1 -> Filterkorrektur_Hardware/1(u)
  theta_el/1 -> Cast To Single/1
  Cast To Single/1 -> Filterkorrektur_Hardware/3("phi ")
  Demux7/1 -> u_d/1
  Demux1/1 -> u_a_corr/1
  Demux1/2 -> u_b_corr/1
  Demux1/3 -> u_c_corr/1

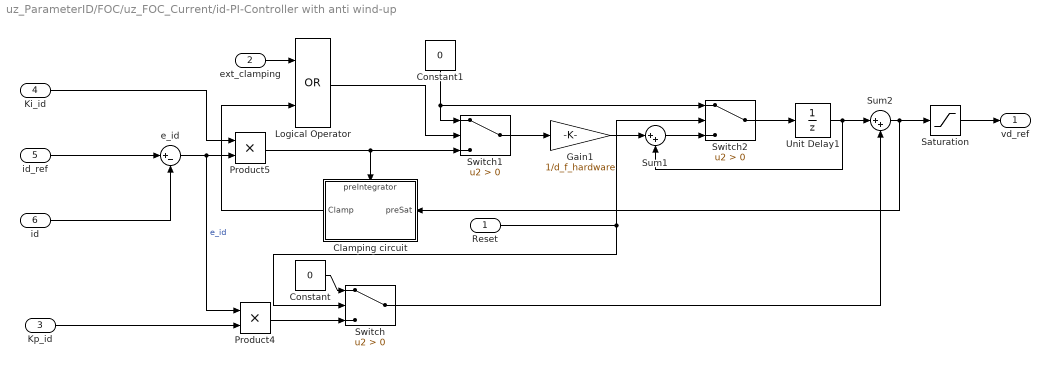
== system uz_ParameterID/FOC/uz_FOC_Current/id-PI-Controller with anti wind-up ==
  Reset : Inport
  ext_clamping : Inport  Port=2
  Kp_id : Inport  Port=3
  Ki_id : Inport  Port=4
  id_ref : Inport  Port=5
  id : Inport  Port=6
  Clamping circuit : Subsystem
      settings: PortSchema="{\"entries\":[{\"content\":{\"sides\":[{\"content\":{\"connectorIds\":[\"In1\"]},\"type\":\"ConnectorPlacement.EquallySpacedRectSide\",\"uuid\":\"9b5eb3d3-336d-4b55-a615-0420b1cf4a48\"},{\"content\":{\"connectorIds\":[\"Out1\"],\"side\":\"RIGHT\"},\"type\":\"ConnectorPlacement.EquallySpacedRectSide\",\"uuid\":\"a73559ab-79dd-4c84-b45a-6a43ba4812e9\"},{\"content\":{\"connectorIds\":[\"In2\"],\"side\":\"TOP\"},\"type\":\"ConnectorPlacement.EquallySpacedRectSide\",\"uuid\":\"82c30f31-c271-4a2b-89be-8686aa9e20f3\"}]},\"type\":\"ConnectorPlacement.EquallySpacedConnector\",\"uuid\":\"376d2fe4-39b3-495b-8d80-8756076e2730\"}],\"packageUris\":[\"http://schema.mathworks.com/mf0/Connector/R2020b\"],\"version\":\"1.0\"}"
  Constant : Constant  Value=0  SampleTime=1/d_f_hardware
  Constant1 : Constant  Value=0  SampleTime=1/d_f_hardware
  Gain1 : Gain  Gain=1/d_f_hardware
  Logical Operator : Logic  Operator=OR  AllPortsSameDT=off  OutDataTypeStr=boolean
  Product4 : Product
  Product5 : Product
  Saturation : Saturate  UpperLimit=d_y_max  LowerLimit=d_y_min
  Sum1 : Sum  Inputs=|++  OutDataTypeStr=single
  Sum2 : Sum  Inputs=|++  OutDataTypeStr=single
  Switch : Switch  Criteria=u2 > Threshold
  Switch1 : Switch  Criteria=u2 > Threshold
  Switch2 : Switch  Criteria=u2 > Threshold
  Unit Delay1 : UnitDelay  SampleTime=-1  HasFrameUpgradeWarning=on
  e_id : Sum  Inputs=|+-
  vd_ref : Outport
  wires:
  Unit Delay1/1 -> Sum2/1, Sum1/2
  Kp_id/1 -> Product4/2
  id_ref/1 -> e_id/1
  Ki_id/1 -> Product5/1
  id/1 -> e_id/2
  e_id/1 -> Product5/2, Product4/1  "e_id"
  Switch/1 -> Sum2/2
  Logical Operator/1 -> Switch1/2
  ext_clamping/1 -> Logical Operator/1
  Sum2/1 -> Saturation/1, Clamping circuit/1(preSat)
  Clamping circuit/1(Clamp) -> Logical Operator/2
  Product5/1 -> Switch1/3, Clamping circuit/2(preIntegrator)
  Saturation/1 -> vd_ref/1
  Constant/1 -> Switch/1
  Product4/1 -> Switch/3
  Gain1/1 -> Sum1/1
  Constant1/1 -> Switch2/1, Switch1/1
  Reset/1 -> Switch/2, Switch2/2
  Sum1/1 -> Switch2/3
  Switch2/1 -> Unit Delay1/1
  Switch1/1 -> Gain1/1

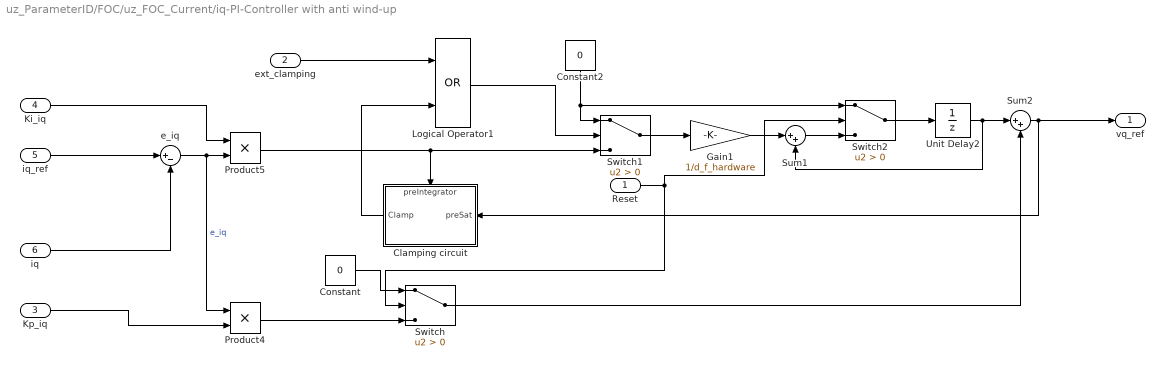
== system uz_ParameterID/FOC/uz_FOC_Current/iq-PI-Controller with anti wind-up ==
  Reset : Inport
  ext_clamping : Inport  Port=2
  Kp_iq : Inport  Port=3
  Ki_iq : Inport  Port=4
  iq_ref : Inport  Port=5
  iq : Inport  Port=6
  Clamping circuit : Subsystem
      settings: PortSchema="{\"entries\":[{\"content\":{\"sides\":[{\"content\":{\"connectorIds\":[\"In1\"]},\"type\":\"ConnectorPlacement.EquallySpacedRectSide\",\"uuid\":\"9b5eb3d3-336d-4b55-a615-0420b1cf4a48\"},{\"content\":{\"connectorIds\":[\"Out1\"],\"side\":\"RIGHT\"},\"type\":\"ConnectorPlacement.EquallySpacedRectSide\",\"uuid\":\"a73559ab-79dd-4c84-b45a-6a43ba4812e9\"},{\"content\":{\"connectorIds\":[\"In2\"],\"side\":\"TOP\"},\"type\":\"ConnectorPlacement.EquallySpacedRectSide\",\"uuid\":\"82c30f31-c271-4a2b-89be-8686aa9e20f3\"}]},\"type\":\"ConnectorPlacement.EquallySpacedConnector\",\"uuid\":\"376d2fe4-39b3-495b-8d80-8756076e2730\"}],\"packageUris\":[\"http://schema.mathworks.com/mf0/Connector/R2020b\"],\"version\":\"1.0\"}"
  Constant : Constant  Value=0  SampleTime=1/d_f_hardware
  Constant2 : Constant  Value=0  SampleTime=1/d_f_hardware
  Gain1 : Gain  Gain=1/d_f_hardware
  Logical Operator1 : Logic  Operator=OR  AllPortsSameDT=off  OutDataTypeStr=boolean
  Product4 : Product
  Product5 : Product
  Sum1 : Sum  Inputs=|++  OutDataTypeStr=single
  Sum2 : Sum  Inputs=|++  OutDataTypeStr=single
  Switch : Switch  Criteria=u2 > Threshold
  Switch1 : Switch  Criteria=u2 > Threshold
  Switch2 : Switch  Criteria=u2 > Threshold
  Unit Delay2 : UnitDelay  SampleTime=-1  HasFrameUpgradeWarning=on
  e_iq : Sum  Inputs=|+-
  vq_ref : Outport
  wires:
  ext_clamping/1 -> Logical Operator1/1
  Kp_iq/1 -> Product4/2
  Ki_iq/1 -> Product5/1
  iq_ref/1 -> e_iq/1
  iq/1 -> e_iq/2
  e_iq/1 -> Product5/2, Product4/1  "e_iq"
  Unit Delay2/1 -> Sum2/1, Sum1/2
  Clamping circuit/1(Clamp) -> Logical Operator1/2
  Sum2/1 -> vq_ref/1, Clamping circuit/1(preSat)
  Switch/1 -> Sum2/2
  Constant/1 -> Switch/1
  Product4/1 -> Switch/3
  Switch2/1 -> Unit Delay2/1
  Gain1/1 -> Sum1/1
  Constant2/1 -> Switch2/1, Switch1/1
  Sum1/1 -> Switch2/3
  Product5/1 -> Switch1/3, Clamping circuit/2(preIntegrator)
  Switch1/1 -> Gain1/1
  Reset/1 -> Switch2/2, Switch/2
  Logical Operator1/1 -> Switch1/2

== system uz_ParameterID/FOC/uz_FOC_Current/linear decouppling ==
  i_q : Inport
  i_d : Inport  Port=2
  omega_el : Inport  Port=3
  Gain : Gain  Gain=-d_L_q
  Gain4 : Gain  Gain=d_L_d
  Product : Product  SaturateOnIntegerOverflow=on
  Product1 : Product  SaturateOnIntegerOverflow=on
  Sum : Sum  Inputs=|++
  d_psi_pm : Constant  Value=d_psi_pm  OutDataTypeStr=Inherit: Inherit via back propagation  SampleTime=1/d_f_hardware
  v_d_decoup : Outport  VectorParamsAs1DForOutWhenUnconnected=off
  v_q_decoup : Outport  Port=2  VectorParamsAs1DForOutWhenUnconnected=off
  wires:
  i_q/1 -> Product/1
  Product1/1 -> v_q_decoup/1
  Gain/1 -> Product/2
  Sum/1 -> Product1/1
  Product/1 -> v_d_decoup/1
  omega_el/1 -> Gain/1, Product1/2
  Gain4/1 -> Sum/1
  d_psi_pm/1 -> Sum/2
  i_d/1 -> Gain4/1

== system uz_ParameterID/FOC/uz_FOC_Speed/Field Weakening ==
  omega_el : Inport  OutDataTypeStr=single
  V_DC : Inport  Port=2  OutDataTypeStr=single
  id_ref_input : Inport  Port=3  OutDataTypeStr=single
  Constant : Constant  Value=d_R_ph  OutDataTypeStr=single
  Constant1 : Constant  Value=d_L_q  OutDataTypeStr=single
  Constant2 : Constant  Value=d_L_d  OutDataTypeStr=single
  Constant3 : Constant  Value=d_psi_pm  OutDataTypeStr=single
  Constant4 : Constant  Value=d_i_max  OutDataTypeStr=single
  MATLAB Function : MATLAB Function  TreatAsAtomicUnit=on
  Saturation : Saturate  UpperLimit=d_i_max  LowerLimit=d_i_min
  iq_max : Outport  OutDataTypeStr=single
  id_Soll : Outport  Port=2  OutDataTypeStr=single
  wires:
  Constant4/1 -> MATLAB Function/1(I_max)
  V_DC/1 -> MATLAB Function/2(V_DC)
  Constant/1 -> MATLAB Function/3(R)
  Constant1/1 -> MATLAB Function/4(Lq)
  Constant2/1 -> MATLAB Function/5(Ld)
  Constant3/1 -> MATLAB Function/6(psi_pm)
  omega_el/1 -> MATLAB Function/7(omega_el)
  MATLAB Function/2(iq_max) -> iq_max/1
  MATLAB Function/1(id_soll) -> id_Soll/1
  id_ref_input/1 -> Saturation/1
  Saturation/1 -> MATLAB Function/8(id_ref_input)

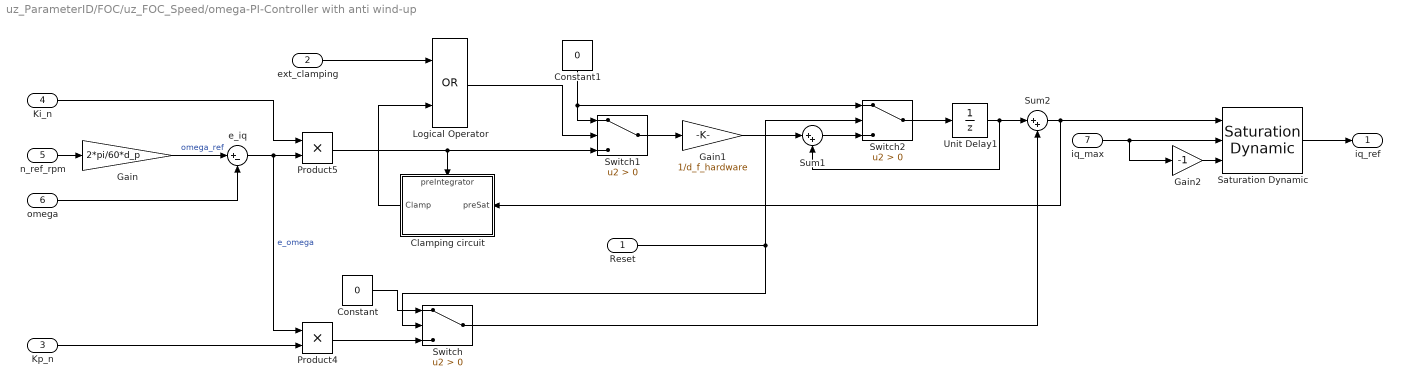
== system uz_ParameterID/FOC/uz_FOC_Speed/omega-PI-Controller with anti wind-up ==
  Reset : Inport
  ext_clamping : Inport  Port=2
  Kp_n : Inport  Port=3
  Ki_n : Inport  Port=4
  n_ref_rpm : Inport  Port=5
  omega : Inport  Port=6
  iq_max : Inport  Port=7
  Clamping circuit : Subsystem
      settings: PortSchema="{\"entries\":[{\"content\":{\"sides\":[{\"content\":{\"connectorIds\":[\"In1\"]},\"type\":\"ConnectorPlacement.EquallySpacedRectSide\",\"uuid\":\"9b5eb3d3-336d-4b55-a615-0420b1cf4a48\"},{\"content\":{\"connectorIds\":[\"Out1\"],\"side\":\"RIGHT\"},\"type\":\"ConnectorPlacement.EquallySpacedRectSide\",\"uuid\":\"a73559ab-79dd-4c84-b45a-6a43ba4812e9\"},{\"content\":{\"connectorIds\":[\"In2\"],\"side\":\"TOP\"},\"type\":\"ConnectorPlacement.EquallySpacedRectSide\",\"uuid\":\"82c30f31-c271-4a2b-89be-8686aa9e20f3\"}]},\"type\":\"ConnectorPlacement.EquallySpacedConnector\",\"uuid\":\"376d2fe4-39b3-495b-8d80-8756076e2730\"}],\"packageUris\":[\"http://schema.mathworks.com/mf0/Connector/R2020b\"],\"version\":\"1.0\"}"
  Constant : Constant  Value=0  SampleTime=1/d_f_hardware
  Constant1 : Constant  Value=0  SampleTime=1/d_f_hardware
  Gain : Gain  Gain=2*pi/60*d_p
  Gain1 : Gain  Gain=1/d_f_hardware
  Gain2 : Gain  Gain=-1
  Logical Operator : Logic  Operator=OR  AllPortsSameDT=off  OutDataTypeStr=boolean
  Product4 : Product
  Product5 : Product
  Saturation Dynamic : simulink/Discontinuities/Saturation Dynamic  OutMin=[]  OutMax=[]  OutDataTypeStr=Inherit: Same as second input  OutDataType=fixdt(1, 16)  OutScaling=2^-10  DoSatur=off
  Sum1 : Sum  Inputs=|++  OutDataTypeStr=single
  Sum2 : Sum  Inputs=|++  OutDataTypeStr=single
  Switch : Switch  Criteria=u2 > Threshold
  Switch1 : Switch  Criteria=u2 > Threshold
  Switch2 : Switch  Criteria=u2 > Threshold
  Unit Delay1 : UnitDelay  SampleTime=-1  HasFrameUpgradeWarning=on
  e_iq : Sum  Inputs=|+-
  iq_ref : Outport
  wires:
  Kp_n/1 -> Product4/2
  Ki_n/1 -> Product5/1
  Gain/1 -> e_iq/1  "omega_ref"
  omega/1 -> e_iq/2
  e_iq/1 -> Product5/2, Product4/1  "e_omega"
  Switch/1 -> Sum2/2
  Unit Delay1/1 -> Sum2/1, Sum1/2
  Sum2/1 -> Saturation Dynamic/1, Clamping circuit/1(preSat)
  ext_clamping/1 -> Logical Operator/1
  Product5/1 -> Switch1/3, Clamping circuit/2(preIntegrator)
  Clamping circuit/1(Clamp) -> Logical Operator/2
  Constant/1 -> Switch/1
  Reset/1 -> Switch/2, Switch2/2
  Product4/1 -> Switch/3
  Constant1/1 -> Switch2/1, Switch1/1
  Logical Operator/1 -> Switch1/2
  n_ref_rpm/1 -> Gain/1
  Switch1/1 -> Gain1/1
  Gain1/1 -> Sum1/1
  Switch2/1 -> Unit Delay1/1
  Sum1/1 -> Switch2/3
  iq_max/1 -> Gain2/1, Saturation Dynamic/2
  Gain2/1 -> Saturation Dynamic/3
  Saturation Dynamic/1 -> iq_ref/1

== system uz_ParameterID/Hardware/Coupling Encoder/Inertia ==
  Trägheitsmoment3 : fl_lib/Mechanical/Rotational Elements/Inertia  Commented=on  inertia=d_J_Coupling_M_E kg*m^2  num_ports=foundation.enum.numPorts2.one  w_specify=off  w_priority=High  w=0 rad/s  w_nominal_specify=off  w_nominal_unit=rad/s  w_nominal_value=1  t_specify=off  t_priority=None  t=0 N*m  t_nominal_specify=off  t_nominal_unit=N*m  t_nominal_value=1
      settings: AttributesFormatString=J in [%<inertia_unit>]
  Input : PMIOPort  Side=Left
  output : PMIOPort  Port=2  Side=Right
  connections:
  Input/RConn1 -- Trägheitsmoment3/LConn1 -- output/RConn1

== system uz_ParameterID/Hardware/Coupling Encoder/Spring Damper System ==
  Rotational Spring : fl_lib/Mechanical/Rotational Elements/Rotational Spring  spr_rate=d_c_Coupling_M_E N*m/rad  w_specify=off  w_priority=None  w=0 rad/s  w_nominal_specify=off  w_nominal_unit=rad/s  w_nominal_value=1  t_specify=off  t_priority=None  t=0 N*m  t_nominal_specify=off  t_nominal_unit=N*m  t_nominal_value=1  phi_specify=off  phi_priority=High  phi=0 rad  phi_nominal_specify=off  phi_nominal_unit=rad  phi_nominal_value=1
  Trägheitsmoment1 : fl_lib/Mechanical/Rotational Elements/Inertia  inertia=d_J_Coupling_M_E/2 kg*m^2  num_ports=foundation.enum.numPorts2.one  w_specify=off  w_priority=High  w=0 rad/s  w_nominal_specify=off  w_nominal_unit=rad/s  w_nominal_value=1  t_specify=off  t_priority=None  t=0 N*m  t_nominal_specify=off  t_nominal_unit=N*m  t_nominal_value=1
      settings: AttributesFormatString=J in [%<inertia_unit>]
  Trägheitsmoment3 : fl_lib/Mechanical/Rotational Elements/Inertia  inertia=d_J_Coupling_M_E/2 kg*m^2  num_ports=foundation.enum.numPorts2.one  w_specify=off  w_priority=High  w=0 rad/s  w_nominal_specify=off  w_nominal_unit=rad/s  w_nominal_value=1  t_specify=off  t_priority=None  t=0 N*m  t_nominal_specify=off  t_nominal_unit=N*m  t_nominal_value=1
      settings: AttributesFormatString=J in [%<inertia_unit>]
  dm : fl_lib/Mechanical/Rotational Elements/Rotational Damper  Commented=on  D=0 N*m/(rad/s)  w_specify=off  w_priority=None  w=0 rad/s  w_nominal_specify=off  w_nominal_unit=rad/s  w_nominal_value=1  t_specify=off  t_priority=None  t=0 N*m  t_nominal_specify=off  t_nominal_unit=N*m  t_nominal_value=1
  Input : PMIOPort  Side=Left
  output : PMIOPort  Port=2  Side=Right
  connections:
  Rotational Spring/LConn1 -- dm/LConn1 -- Input/RConn1 -- Trägheitsmoment3/LConn1
  Trägheitsmoment1/LConn1 -- Rotational Spring/RConn1 -- dm/RConn1 -- output/RConn1

== system uz_ParameterID/Hardware/Measurement Shaft/Spring Damper System ==
  Rotational Spring : fl_lib/Mechanical/Rotational Elements/Rotational Spring  spr_rate=d_c_Ms N*m/rad  w_specify=off  w_priority=None  w=0 rad/s  w_nominal_specify=off  w_nominal_unit=rad/s  w_nominal_value=1  t_specify=off  t_priority=None  t=0 N*m  t_nominal_specify=off  t_nominal_unit=N*m  t_nominal_value=1  phi_specify=off  phi_priority=High  phi=0 rad  phi_nominal_specify=off  phi_nominal_unit=rad  phi_nominal_value=1
  Trägheitsmoment1 : fl_lib/Mechanical/Rotational Elements/Inertia  inertia=d_J_Ms_L kg*m^2  num_ports=foundation.enum.numPorts2.one  w_specify=off  w_priority=High  w=0 rad/s  w_nominal_specify=off  w_nominal_unit=rad/s  w_nominal_value=1  t_specify=off  t_priority=None  t=0 N*m  t_nominal_specify=off  t_nominal_unit=N*m  t_nominal_value=1
      settings: AttributesFormatString=J in [%<inertia_unit>]
  Trägheitsmoment3 : fl_lib/Mechanical/Rotational Elements/Inertia  inertia=d_J_Ms_M kg*m^2  num_ports=foundation.enum.numPorts2.one  w_specify=off  w_priority=High  w=0 rad/s  w_nominal_specify=off  w_nominal_unit=rad/s  w_nominal_value=1  t_specify=off  t_priority=None  t=0 N*m  t_nominal_specify=off  t_nominal_unit=N*m  t_nominal_value=1
      settings: AttributesFormatString=J in [%<inertia_unit>]
  dm : fl_lib/Mechanical/Rotational Elements/Rotational Damper  D=d_d_TMS N*m/(rad/s)  w_specify=off  w_priority=None  w=0 rad/s  w_nominal_specify=off  w_nominal_unit=rad/s  w_nominal_value=1  t_specify=off  t_priority=None  t=0 N*m  t_nominal_specify=off  t_nominal_unit=N*m  t_nominal_value=1
  Input : PMIOPort  Side=Left
  output : PMIOPort  Port=2  Side=Right
  connections:
  Rotational Spring/LConn1 -- dm/LConn1 -- Trägheitsmoment3/LConn1 -- Input/RConn1
  Rotational Spring/RConn1 -- dm/RConn1 -- output/RConn1 -- Trägheitsmoment1/LConn1

== system uz_ParameterID/Hardware/Measurement Shaft/default ==
  Trägheitsmoment3 : fl_lib/Mechanical/Rotational Elements/Inertia  inertia=d_J_Ms_M+d_J_Ms_L kg*m^2  num_ports=foundation.enum.numPorts2.one  w_specify=off  w_priority=High  w=0 rad/s  w_nominal_specify=off  w_nominal_unit=rad/s  w_nominal_value=1  t_specify=off  t_priority=None  t=0 N*m  t_nominal_specify=off  t_nominal_unit=N*m  t_nominal_value=1
      settings: AttributesFormatString=J in [%<inertia_unit>]
  Input : PMIOPort  Side=Left
  output : PMIOPort  Port=2  Side=Right
  connections:
  Trägheitsmoment3/LConn1 -- output/RConn1 -- Input/RConn1
